simulink library "IOBlock_Library_TTC580"  (R2021a)
settings: Solver=ode45  StartTime=0.0  StopTime=10.0  RelTol=1e-3
PreLoadFcn:
  | addpath(genpath(fileparts(which('IOBlock_Library_TTC580'))));
  | %addpath(genpath(fileparts(which('IOBlock_Library_TTC580.mdl'))))
  | try
  | addpath(genpath([fileparts(which('IOBlock_Library_TTC580')),'\..\DBC_Importer']));
  | addpath(genpath([fileparts(which('IOBlock_Library_TTC580')),'\..\EEPROM_Importer']));
  | addpath(genpath([fileparts(which('IOBlock_Library_TTC580')),'\..\UserDoc']));
  | catch
  | warning('IOBlock_Library_TTC580: add path to DBC_Importer and EEPROM_Importer manually');
  | end
  | try
  | if exist('..\CustomPackage\scripts\OpenAllPackages.m','file')
  |      run('..\CustomPackage\scripts\OpenAllPackages.m'); %always available, ggf. empty
  | end
  | catch
  | warning('A problem occurred opening automatically the CustomPackage. Please open libraries manually');
  | end
  | try
  | set_param(0,'EditorSmartEditingHotParam','off');
  | catch
  | warning('Simlink preferences for ''Edit key parameter when adding new blocks'' needs to be unchecked manually');
  | end
undefined symbols (not defined in the file or in its folder): ADC_Absolute_10V, ADC_Absolute_32V, ADC_Absolute_5V, ADC_BoardTemp, ADC_ChannelInit, ADC_Current, ADC_Get, ADC_K15_, ADC_Ratiometric_10V, ADC_Ratiometric_5V, ADC_Resistive, ADC_SensorSupply, ADC_UBAT, bit_packing, bit_unpacking, CAN_ConfigMsg, compare2error, compare2FET_PROT_REENABLE, crc32_calc_intern, CRC32_EEPROM_Read, CRC32_EEPROM_Write, DIAG_EnterSafestate, DIAG_Status, DIAG_Status_internal, EEPROM_Mirror, EEPROM_Read, EEPROM_Read_OffsetIn, EEPROM_Read_Raw, EEPROM_Write, EEPROM_Write_OffsetIn, EEPROM_Write_Raw, EnterSafestate, FPU_Handler, Get_DI, Get_DI_VarThreshold, Get_K15_, Get_Pulse_Freq_Curr, Get_Pulse_Freq_Volt, Get_WakeUp, GetDateAndTime, IO_ADC_ResetProtection, IO_Blk_Lib_TTC500, IO_CAN_ReadMsg, IO_CAN_WriteMsg, IO_DI_Get, IO_DI_Init, IO_DI_Init_Var, IO_DO_GetCur, IO_DO_GetVoltage, IO_DO_Init, IO_DO_ResetProtection, IO_DO_Set, IO_Driver_GetSerialNumber, IO_Driver_GetVersionOfDriver, IO_Driver_GetVersionOfFPGA, IO_EEPROM_GetStatus, IO_EEPROM_Init, IO_EEPROM_Read_raw, IO_EEPROM_Write, IO_EEPROM_Write_OffsetIn ... (+73)
libraries: simulink x43
(part 16 of 18)

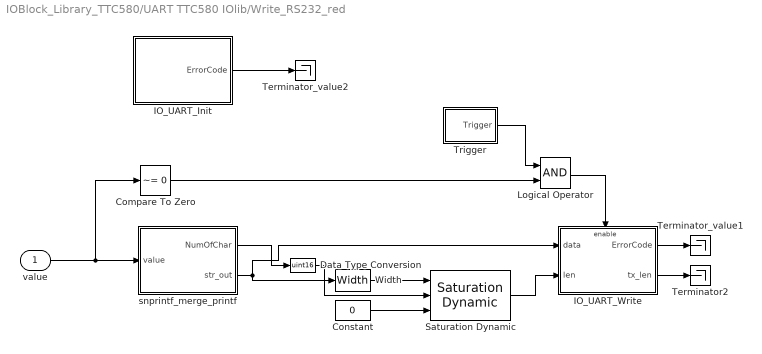
== system IOBlock_Library_TTC580/UART TTC580 IOlib/Write_RS232_red ==
  value : Inport
  Compare To Zero : simulink/Logic and Bit Operations/Compare To Zero  relop=~=  OutDataTypeStr=boolean
  Constant : Constant  Value=0  OutDataTypeStr=uint16
  Data Type Conversion : DataTypeConversion  OutDataTypeStr=uint16
  IO_UART_Init : Subsystem  LoadFcn=|  mask(IO_UART_Init_Code){SampleTime=-1, ttlib=IO_Blk_Lib_TTC500, ttDescription=IO_UART_Init, tt_iolib_version=0.25, baudrate=115200, dbits='8', par='IO_UART_PARITY_NONE', sbits='1'}
      | try
      | %
      | %Upgrade Information - standard BEGIN
      | new_color = 'blue';
      | new_ver = '0.25';
      | act_ver = get_param(gcb,'tt_iolib_version');
      | if not(strcmp(act_ver,new_ver))
      |     disp(['Upgrade block: ',gcb,char(10),'       Version: ',act_ver,' to ',new_ver]);
      |     %switch - case for specific upgrade information e.g. additional parameter required 
      |     %Change appearance and version information
      |     set_param(gcb,'ForegroundColor',new_color);
      |     set_param(gcb,'tt_iolib_version',new_ver);
      | end
      | %Upgrade Information - standard END
      | catch
      | %Standard catch section BEGIN
      | errordlg('An error occurred in a callback of the TTC580-BlockLib. Please open the Diagnostic Viewer for further details');
      | disp(' ');
      | disp('------------------------------------------------------------');
      | disp('An error occurred in a callback of the TTC580-BlockLib.');
      | disp(['Please check the parameters in the mask of ',gcb]);
      | disp('If you do not encounter any violations, then please '); 
      | disp('copy the following lines and report this to support@ttcontrol.com ');
      | disp('<< begin of error message dump >>');
      | disp(['Version of TTC580-BlockLib: ', get_param(gcb,'tt_iolib_version')]);
      | disp(get_param(gcb,'ttDescription'));
      | disp(gcb);
      | x=lasterror;disp(x.message);
      | disp(get_param(gcb,'MaskValues'));
      | disp(version);
      | disp(computer);
      | disp('<< end of error message dump >>');
      | disp('------------------------------------------------------------');
      | disp(' ');
      | %Standard catch section END
      | end
      mask help: Initialization of the UART communication driver.
      mask init:
      | %
      settings: CopyFcn=%deleted
      mask Help: No further help available for this block
      mask Callback baudrate: %
      mask Callback dbits: %
      mask Callback par: %
      mask Callback sbits: %
  IO_UART_Write : Subsystem  LoadFcn=|  mask(IO_UART_Write_Code){SampleTime=-1, ttlib=IO_Blk_Lib_TTC500, ttDescription=IO_UART_Write, tt_iolib_version=0.25}
      | try
      | %
      | %Upgrade Information - standard BEGIN
      | new_color = 'blue';
      | new_ver = '0.25';
      | act_ver = get_param(gcb,'tt_iolib_version');
      | if not(strcmp(act_ver,new_ver))
      |     disp(['Upgrade block: ',gcb,char(10),'       Version: ',act_ver,' to ',new_ver]);
      |     %switch - case for specific upgrade information e.g. additional parameter required 
      |     %Change appearance and version information
      |     set_param(gcb,'ForegroundColor',new_color);
      |     set_param(gcb,'tt_iolib_version',new_ver);
      | end
      | %Upgrade Information - standard END
      | catch
      | %Standard catch section BEGIN
      | errordlg('An error occurred in a callback of the TTC580-BlockLib. Please open the Diagnostic Viewer for further details');
      | disp(' ');
      | disp('------------------------------------------------------------');
      | disp('An error occurred in a callback of the TTC580-BlockLib.');
      | disp(['Please check the parameters in the mask of ',gcb]);
      | disp('If you do not encounter any violations, then please '); 
      | disp('copy the following lines and report this to support@ttcontrol.com ');
      | disp('<< begin of error message dump >>');
      | disp(['Version of TTC580-BlockLib: ', get_param(gcb,'tt_iolib_version')]);
      | disp(get_param(gcb,'ttDescription'));
      | disp(gcb);
      | x=lasterror;disp(x.message);
      | disp(get_param(gcb,'MaskValues'));
      | disp(version);
      | disp(computer);
      | disp('<< end of error message dump >>');
      | disp('------------------------------------------------------------');
      | disp(' ');
      | %Standard catch section END
      | end
      mask help: Write data to serial interface.
      mask init:
      | %
      settings: CopyFcn=%deleted  RTWSystemCode=Inline
      mask Help: No further help available for this block
  Logical Operator : Logic  AllPortsSameDT=off  OutDataTypeStr=boolean
  Saturation Dynamic : simulink/Discontinuities/Saturation Dynamic  OutMin=[]  OutMax=[]  OutDataTypeStr=uint16  OutputDataTypeScalingMode=uint16  OutDataType=fixdt(1, 16)  OutScaling=2^-10  DoSatur=off
  Terminator2 : Terminator
  Terminator_value1 : Terminator
  Terminator_value2 : Terminator
  Trigger : Subsystem  mask(Derate Trigger){derate=derate_val}
      mask help: derate "n": every n-th cylce a trigger is submitted
  Width : Width  DataType=uint16
  snprintf_merge_printf : Subsystem  LoadFcn=|  mask(snprintf_merge_printf_Code){SampleTime=-1, ttlib=IO_Blk_Lib_TTC500, ttDescription=snprintf_merge_printf, tt_iolib_version=0.25, max_size=80, Comment=['\033[0;31m',Comment,'\033[0m']}
      | try
      | %
      | %Upgrade Information - standard BEGIN
      | new_color = 'blue';
      | new_ver = '0.25';
      | act_ver = get_param(gcb,'tt_iolib_version');
      | if not(strcmp(act_ver,new_ver))
      |     disp(['Upgrade block: ',gcb,char(10),'       Version: ',act_ver,' to ',new_ver]);
      |     %switch - case for specific upgrade information e.g. additional parameter required 
      |     %Change appearance and version information
      |     set_param(gcb,'ForegroundColor',new_color);
      |     set_param(gcb,'tt_iolib_version',new_ver);
      | end
      | %Upgrade Information - standard END
      | catch
      | %Standard catch section BEGIN
      | errordlg('An error occurred in a callback of the TTC580-BlockLib. Please open the Diagnostic Viewer for further details');
      | disp(' ');
      | disp('------------------------------------------------------------');
      | disp('An error occurred in a callback of the TTC580-BlockLib.');
      | disp(['Please check the parameters in the mask of ',gcb]);
      | disp('If you do not encounter any violations, then please '); 
      | disp('copy the following lines and report this to support@ttcontrol.com ');
      | disp('<< begin of error message dump >>');
      | disp(['Version of TTC580-BlockLib: ', get_param(gcb,'tt_iolib_version')]);
      | disp(get_param(gcb,'ttDescription'));
      | disp(gcb);
      | x=lasterror;disp(x.message);
      | disp(get_param(gcb,'MaskValues'));
      | disp(version);
      | disp(computer);
      | disp('<< end of error message dump >>');
      | disp('------------------------------------------------------------');
      | disp(' ');
      | %Standard catch section END
      | end
      mask help:
      | The C library function snprintf sends formatted output to a string with maximum length of n characters.
      | This snprintf implementation adds LF and reset cursor information the way that the printf implementation did it before
      mask init:
      | %
      settings: CopyFcn=%deleted
      mask Help: No further help available for this block
      mask Callback max_size: %
      mask Callback Comment: %
  wires:
  Data Type Conversion/1 -> Saturation Dynamic/2
  IO_UART_Write/1(ErrorCode) -> Terminator_value1/1
  Constant/1 -> Saturation Dynamic/3
  value/1 -> snprintf_merge_printf/1(value), Compare To Zero/1
  snprintf_merge_printf/1(NumOfChar) -> Data Type Conversion/1
  Width/1 -> Saturation Dynamic/1
  IO_UART_Init/1(ErrorCode) -> Terminator_value2/1
  Saturation Dynamic/1 -> IO_UART_Write/2(len)
  snprintf_merge_printf/2(str_out) -> IO_UART_Write/1(data), Width/1
  IO_UART_Write/2(tx_len) -> Terminator2/1
  Trigger/1(Trigger) -> Logical Operator/1
  Compare To Zero/1 -> Logical Operator/2
  Logical Operator/1 -> IO_UART_Write/Enable

== system IOBlock_Library_TTC580/ADC Blocks TTC580 IOlib/ADC_Absolute_10V/ADC_ChannelInit ==
  ADC_ChannelInit_s : S-Function  FunctionName=ADC_ChannelInit_s  Parameters=SampleTime,adc_channel,adc_type,range,pupd,sensor_supply,safety_conf  SFunctionDeploymentMode=off  EnableBusSupport=off
  ErrorCode : Outport  VectorParamsAs1DForOutWhenUnconnected=off
  wires:
  ADC_ChannelInit_s/1 -> ErrorCode/1

== system IOBlock_Library_TTC580/ADC Blocks TTC580 IOlib/ADC_Absolute_10V/ADC_Get ==
  ADC_Get_s : S-Function  FunctionName=ADC_Get_s  Parameters=SampleTime,adc_channel  SFunctionDeploymentMode=off  EnableBusSupport=off
  ErrorCode : Outport  VectorParamsAs1DForOutWhenUnconnected=off
  adc_value : Outport  Port=2  VectorParamsAs1DForOutWhenUnconnected=off
  fresh : Outport  Port=3  VectorParamsAs1DForOutWhenUnconnected=off
  wires:
  ADC_Get_s/3 -> fresh/1
  ADC_Get_s/2 -> adc_value/1
  ADC_Get_s/1 -> ErrorCode/1

== system IOBlock_Library_TTC580/ADC Blocks TTC580 IOlib/ADC_Absolute_32V/ADC_ChannelInit ==
  ADC_ChannelInit_s : S-Function  FunctionName=ADC_ChannelInit_s  Parameters=SampleTime,adc_channel,adc_type,range,pupd,sensor_supply,safety_conf  SFunctionDeploymentMode=off  EnableBusSupport=off
  ErrorCode : Outport  VectorParamsAs1DForOutWhenUnconnected=off
  wires:
  ADC_ChannelInit_s/1 -> ErrorCode/1

== system IOBlock_Library_TTC580/ADC Blocks TTC580 IOlib/ADC_Absolute_32V/ADC_Get ==
  ADC_Get_s : S-Function  FunctionName=ADC_Get_s  Parameters=SampleTime,adc_channel  SFunctionDeploymentMode=off  EnableBusSupport=off
  ErrorCode : Outport  VectorParamsAs1DForOutWhenUnconnected=off
  adc_value : Outport  Port=2  VectorParamsAs1DForOutWhenUnconnected=off
  fresh : Outport  Port=3  VectorParamsAs1DForOutWhenUnconnected=off
  wires:
  ADC_Get_s/3 -> fresh/1
  ADC_Get_s/2 -> adc_value/1
  ADC_Get_s/1 -> ErrorCode/1

== system IOBlock_Library_TTC580/ADC Blocks TTC580 IOlib/ADC_Absolute_5V/ADC_ChannelInit ==
  ADC_ChannelInit_s : S-Function  FunctionName=ADC_ChannelInit_s  Parameters=SampleTime,adc_channel,adc_type,range,pupd,sensor_supply,safety_conf  SFunctionDeploymentMode=off  EnableBusSupport=off
  ErrorCode : Outport  VectorParamsAs1DForOutWhenUnconnected=off
  wires:
  ADC_ChannelInit_s/1 -> ErrorCode/1

== system IOBlock_Library_TTC580/ADC Blocks TTC580 IOlib/ADC_Absolute_5V/ADC_Get ==
  ADC_Get_s : S-Function  FunctionName=ADC_Get_s  Parameters=SampleTime,adc_channel  SFunctionDeploymentMode=off  EnableBusSupport=off
  ErrorCode : Outport  VectorParamsAs1DForOutWhenUnconnected=off
  adc_value : Outport  Port=2  VectorParamsAs1DForOutWhenUnconnected=off
  fresh : Outport  Port=3  VectorParamsAs1DForOutWhenUnconnected=off
  wires:
  ADC_Get_s/3 -> fresh/1
  ADC_Get_s/2 -> adc_value/1
  ADC_Get_s/1 -> ErrorCode/1

== system IOBlock_Library_TTC580/ADC Blocks TTC580 IOlib/ADC_BoardTemp/ADC_ChannelInit ==
  ADC_ChannelInit_s : S-Function  FunctionName=ADC_ChannelInit_s  Parameters=SampleTime,adc_channel,adc_type,range,pupd,sensor_supply,safety_conf  SFunctionDeploymentMode=off  EnableBusSupport=off
  ErrorCode : Outport  VectorParamsAs1DForOutWhenUnconnected=off
  wires:
  ADC_ChannelInit_s/1 -> ErrorCode/1

== system IOBlock_Library_TTC580/ADC Blocks TTC580 IOlib/ADC_BoardTemp/ADC_Get ==
  ADC_Get_s : S-Function  FunctionName=ADC_Get_s  Parameters=SampleTime,adc_channel  SFunctionDeploymentMode=off  EnableBusSupport=off
  ErrorCode : Outport  VectorParamsAs1DForOutWhenUnconnected=off
  adc_value : Outport  Port=2  VectorParamsAs1DForOutWhenUnconnected=off
  fresh : Outport  Port=3  VectorParamsAs1DForOutWhenUnconnected=off
  wires:
  ADC_Get_s/1 -> ErrorCode/1
  ADC_Get_s/2 -> adc_value/1
  ADC_Get_s/3 -> fresh/1

== system IOBlock_Library_TTC580/ADC Blocks TTC580 IOlib/ADC_Current/ADC_ChannelInit ==
  ADC_ChannelInit_s : S-Function  FunctionName=ADC_ChannelInit_s  Parameters=SampleTime,adc_channel,adc_type,range,pupd,sensor_supply,safety_conf  SFunctionDeploymentMode=off  EnableBusSupport=off
  ErrorCode : Outport  VectorParamsAs1DForOutWhenUnconnected=off
  wires:
  ADC_ChannelInit_s/1 -> ErrorCode/1

== system IOBlock_Library_TTC580/ADC Blocks TTC580 IOlib/ADC_Current/ADC_Get ==
  ADC_Get_s : S-Function  FunctionName=ADC_Get_s  Parameters=SampleTime,adc_channel  SFunctionDeploymentMode=off  EnableBusSupport=off
  ErrorCode : Outport  VectorParamsAs1DForOutWhenUnconnected=off
  adc_value : Outport  Port=2  VectorParamsAs1DForOutWhenUnconnected=off
  fresh : Outport  Port=3  VectorParamsAs1DForOutWhenUnconnected=off
  wires:
  ADC_Get_s/3 -> fresh/1
  ADC_Get_s/2 -> adc_value/1
  ADC_Get_s/1 -> ErrorCode/1

== system IOBlock_Library_TTC580/ADC Blocks TTC580 IOlib/ADC_Current/IO_ADC_ResetProtection ==
  Trigger : TriggerPort  VariantControl=(inherit)
  IO_ADC_ResetProtection_s : S-Function  FunctionName=IO_ADC_ResetProtection_s  Parameters=SampleTime,adc_channel  SFunctionDeploymentMode=off  EnableBusSupport=off
  ErrorCode : Outport  VectorParamsAs1DForOutWhenUnconnected=off
  reset_cnt : Outport  Port=2  VectorParamsAs1DForOutWhenUnconnected=off
  wires:
  IO_ADC_ResetProtection_s/2 -> reset_cnt/1
  IO_ADC_ResetProtection_s/1 -> ErrorCode/1

== system IOBlock_Library_TTC580/ADC Blocks TTC580 IOlib/ADC_Current/compare2FET_PROT_REENABLE ==
  Errorcode : Inport  OutDataTypeStr=uint16
  compare2error_s : S-Function  FunctionName=compare2error_s  Parameters=SampleTime,define  SFunctionDeploymentMode=off  EnableBusSupport=off
  b_compare : Outport  VectorParamsAs1DForOutWhenUnconnected=off
  wires:
  Errorcode/1 -> compare2error_s/1
  compare2error_s/1 -> b_compare/1

== system IOBlock_Library_TTC580/ADC Blocks TTC580 IOlib/ADC_K15_/ADC_ChannelInit ==
  ADC_ChannelInit_s : S-Function  FunctionName=ADC_ChannelInit_s  Parameters=SampleTime,adc_channel,adc_type,range,pupd,sensor_supply,safety_conf  SFunctionDeploymentMode=off  EnableBusSupport=off
  ErrorCode : Outport  VectorParamsAs1DForOutWhenUnconnected=off
  wires:
  ADC_ChannelInit_s/1 -> ErrorCode/1

== system IOBlock_Library_TTC580/ADC Blocks TTC580 IOlib/ADC_K15_/ADC_Get ==
  ADC_Get_s : S-Function  FunctionName=ADC_Get_s  Parameters=SampleTime,adc_channel  SFunctionDeploymentMode=off  EnableBusSupport=off
  ErrorCode : Outport  VectorParamsAs1DForOutWhenUnconnected=off
  adc_value : Outport  Port=2  VectorParamsAs1DForOutWhenUnconnected=off
  fresh : Outport  Port=3  VectorParamsAs1DForOutWhenUnconnected=off
  wires:
  ADC_Get_s/1 -> ErrorCode/1
  ADC_Get_s/2 -> adc_value/1
  ADC_Get_s/3 -> fresh/1

== system IOBlock_Library_TTC580/ADC Blocks TTC580 IOlib/ADC_Ratiometric_10V/ADC_ChannelInit ==
  ADC_ChannelInit_s : S-Function  FunctionName=ADC_ChannelInit_s  Parameters=SampleTime,adc_channel,adc_type,range,pupd,sensor_supply,safety_conf  SFunctionDeploymentMode=off  EnableBusSupport=off
  ErrorCode : Outport  VectorParamsAs1DForOutWhenUnconnected=off
  wires:
  ADC_ChannelInit_s/1 -> ErrorCode/1

== system IOBlock_Library_TTC580/ADC Blocks TTC580 IOlib/ADC_Ratiometric_10V/ADC_Get ==
  ADC_Get_s : S-Function  FunctionName=ADC_Get_s  Parameters=SampleTime,adc_channel  SFunctionDeploymentMode=off  EnableBusSupport=off
  ErrorCode : Outport  VectorParamsAs1DForOutWhenUnconnected=off
  adc_value : Outport  Port=2  VectorParamsAs1DForOutWhenUnconnected=off
  fresh : Outport  Port=3  VectorParamsAs1DForOutWhenUnconnected=off
  wires:
  ADC_Get_s/1 -> ErrorCode/1
  ADC_Get_s/2 -> adc_value/1
  ADC_Get_s/3 -> fresh/1

== system IOBlock_Library_TTC580/ADC Blocks TTC580 IOlib/ADC_Ratiometric_10V/POWER_Set_Init ==
  POWER_Set_Init_s : S-Function  FunctionName=POWER_Set_Init_s  Parameters=SampleTime,pin,mode  SFunctionDeploymentMode=off  EnableBusSupport=off
  ErrorCode : Outport  VectorParamsAs1DForOutWhenUnconnected=off
  wires:
  POWER_Set_Init_s/1 -> ErrorCode/1

== system IOBlock_Library_TTC580/ADC Blocks TTC580 IOlib/ADC_Ratiometric_5V/ADC_ChannelInit ==
  ADC_ChannelInit_s : S-Function  FunctionName=ADC_ChannelInit_s  Parameters=SampleTime,adc_channel,adc_type,range,pupd,sensor_supply,safety_conf  SFunctionDeploymentMode=off  EnableBusSupport=off
  ErrorCode : Outport  VectorParamsAs1DForOutWhenUnconnected=off
  wires:
  ADC_ChannelInit_s/1 -> ErrorCode/1

== system IOBlock_Library_TTC580/ADC Blocks TTC580 IOlib/ADC_Ratiometric_5V/ADC_Get ==
  ADC_Get_s : S-Function  FunctionName=ADC_Get_s  Parameters=SampleTime,adc_channel  SFunctionDeploymentMode=off  EnableBusSupport=off
  ErrorCode : Outport  VectorParamsAs1DForOutWhenUnconnected=off
  adc_value : Outport  Port=2  VectorParamsAs1DForOutWhenUnconnected=off
  fresh : Outport  Port=3  VectorParamsAs1DForOutWhenUnconnected=off
  wires:
  ADC_Get_s/1 -> ErrorCode/1
  ADC_Get_s/2 -> adc_value/1
  ADC_Get_s/3 -> fresh/1

== system IOBlock_Library_TTC580/ADC Blocks TTC580 IOlib/ADC_Ratiometric_5V/POWER_Set_Init ==
  POWER_Set_Init_s : S-Function  FunctionName=POWER_Set_Init_s  Parameters=SampleTime,pin,mode  SFunctionDeploymentMode=off  EnableBusSupport=off
  ErrorCode : Outport  VectorParamsAs1DForOutWhenUnconnected=off
  wires:
  POWER_Set_Init_s/1 -> ErrorCode/1

== system IOBlock_Library_TTC580/ADC Blocks TTC580 IOlib/ADC_Resistive/ADC_ChannelInit ==
  ADC_ChannelInit_s : S-Function  FunctionName=ADC_ChannelInit_s  Parameters=SampleTime,adc_channel,adc_type,range,pupd,sensor_supply,safety_conf  SFunctionDeploymentMode=off  EnableBusSupport=off
  ErrorCode : Outport  VectorParamsAs1DForOutWhenUnconnected=off
  wires:
  ADC_ChannelInit_s/1 -> ErrorCode/1

== system IOBlock_Library_TTC580/ADC Blocks TTC580 IOlib/ADC_Resistive/ADC_Get ==
  ADC_Get_s : S-Function  FunctionName=ADC_Get_s  Parameters=SampleTime,adc_channel  SFunctionDeploymentMode=off  EnableBusSupport=off
  ErrorCode : Outport  VectorParamsAs1DForOutWhenUnconnected=off
  adc_value : Outport  Port=2  VectorParamsAs1DForOutWhenUnconnected=off
  fresh : Outport  Port=3  VectorParamsAs1DForOutWhenUnconnected=off
  wires:
  ADC_Get_s/3 -> fresh/1
  ADC_Get_s/2 -> adc_value/1
  ADC_Get_s/1 -> ErrorCode/1

== system IOBlock_Library_TTC580/ADC Blocks TTC580 IOlib/ADC_SensorSupply/ADC_ChannelInit ==
  ADC_ChannelInit_s : S-Function  FunctionName=ADC_ChannelInit_s  Parameters=SampleTime,adc_channel,adc_type,range,pupd,sensor_supply,safety_conf  SFunctionDeploymentMode=off  EnableBusSupport=off
  ErrorCode : Outport  VectorParamsAs1DForOutWhenUnconnected=off
  wires:
  ADC_ChannelInit_s/1 -> ErrorCode/1

== system IOBlock_Library_TTC580/ADC Blocks TTC580 IOlib/ADC_SensorSupply/ADC_Get ==
  ADC_Get_s : S-Function  FunctionName=ADC_Get_s  Parameters=SampleTime,adc_channel  SFunctionDeploymentMode=off  EnableBusSupport=off
  ErrorCode : Outport  VectorParamsAs1DForOutWhenUnconnected=off
  adc_value : Outport  Port=2  VectorParamsAs1DForOutWhenUnconnected=off
  fresh : Outport  Port=3  VectorParamsAs1DForOutWhenUnconnected=off
  wires:
  ADC_Get_s/3 -> fresh/1
  ADC_Get_s/2 -> adc_value/1
  ADC_Get_s/1 -> ErrorCode/1

== system IOBlock_Library_TTC580/ADC Blocks TTC580 IOlib/ADC_UBAT/ADC_ChannelInit ==
  ADC_ChannelInit_s : S-Function  FunctionName=ADC_ChannelInit_s  Parameters=SampleTime,adc_channel,adc_type,range,pupd,sensor_supply,safety_conf  SFunctionDeploymentMode=off  EnableBusSupport=off
  ErrorCode : Outport  VectorParamsAs1DForOutWhenUnconnected=off
  wires:
  ADC_ChannelInit_s/1 -> ErrorCode/1

== system IOBlock_Library_TTC580/ADC Blocks TTC580 IOlib/ADC_UBAT/ADC_Get ==
  ADC_Get_s : S-Function  FunctionName=ADC_Get_s  Parameters=SampleTime,adc_channel  SFunctionDeploymentMode=off  EnableBusSupport=off
  ErrorCode : Outport  VectorParamsAs1DForOutWhenUnconnected=off
  adc_value : Outport  Port=2  VectorParamsAs1DForOutWhenUnconnected=off
  fresh : Outport  Port=3  VectorParamsAs1DForOutWhenUnconnected=off
  wires:
  ADC_Get_s/3 -> fresh/1
  ADC_Get_s/2 -> adc_value/1
  ADC_Get_s/1 -> ErrorCode/1

== system IOBlock_Library_TTC580/CAN  Blocks TTC580 IOlib/ReadMsg_CAN/CAN_ConfigMsg ==
  CAN_ConfigMsg_s : S-Function  FunctionName=CAN_ConfigMsg_s  Parameters=SampleTime,channel,mode,id_format,id,ac_mask  SFunctionDeploymentMode=off  EnableBusSupport=off
  ErrorCode : Outport  VectorParamsAs1DForOutWhenUnconnected=off
  handle : Outport  Port=2  VectorParamsAs1DForOutWhenUnconnected=off
  wires:
  CAN_ConfigMsg_s/2 -> handle/1
  CAN_ConfigMsg_s/1 -> ErrorCode/1

== system IOBlock_Library_TTC580/CAN  Blocks TTC580 IOlib/ReadMsg_CAN/IO_CAN_ReadMsg ==
  handle : Inport
  IO_CAN_ReadMsg_s : S-Function  FunctionName=IO_CAN_ReadMsg_s  Parameters=SampleTime  SFunctionDeploymentMode=off  EnableBusSupport=off
  ErrorCode : Outport  VectorParamsAs1DForOutWhenUnconnected=off
  buffer_data : Outport  Port=2  VectorParamsAs1DForOutWhenUnconnected=off
  buffer_length : Outport  Port=3  VectorParamsAs1DForOutWhenUnconnected=off
  buffer_id_format : Outport  Port=4  VectorParamsAs1DForOutWhenUnconnected=off
  buffer_id : Outport  Port=5  VectorParamsAs1DForOutWhenUnconnected=off
  wires:
  IO_CAN_ReadMsg_s/5 -> buffer_id/1
  IO_CAN_ReadMsg_s/4 -> buffer_id_format/1
  IO_CAN_ReadMsg_s/3 -> buffer_length/1
  IO_CAN_ReadMsg_s/2 -> buffer_data/1
  IO_CAN_ReadMsg_s/1 -> ErrorCode/1
  handle/1 -> IO_CAN_ReadMsg_s/1

== system IOBlock_Library_TTC580/CAN  Blocks TTC580 IOlib/ReadMsg_CAN_derated/CAN_ConfigMsg ==
  CAN_ConfigMsg_s : S-Function  FunctionName=CAN_ConfigMsg_s  Parameters=SampleTime,channel,mode,id_format,id,ac_mask  SFunctionDeploymentMode=off  EnableBusSupport=off
  ErrorCode : Outport  VectorParamsAs1DForOutWhenUnconnected=off
  handle : Outport  Port=2  VectorParamsAs1DForOutWhenUnconnected=off
  wires:
  CAN_ConfigMsg_s/1 -> ErrorCode/1
  CAN_ConfigMsg_s/2 -> handle/1

== system IOBlock_Library_TTC580/CAN  Blocks TTC580 IOlib/ReadMsg_CAN_derated/IO_CAN_ReadMsg_x ==
  handle : Inport
  Enable : EnablePort
  IO_CAN_ReadMsg_s : S-Function  FunctionName=IO_CAN_ReadMsg_s  Parameters=SampleTime  SFunctionDeploymentMode=off  EnableBusSupport=off
  debounce_alternate : Subsystem
  ErrorCode : Outport  InitialOutput=16 %IO_E_STARTUP, just in case not debounced correctly  VectorParamsAs1DForOutWhenUnconnected=off
  buffer_data : Outport  Port=2  VectorParamsAs1DForOutWhenUnconnected=off
  buffer_length : Outport  Port=3  VectorParamsAs1DForOutWhenUnconnected=off
  buffer_id_format : Outport  Port=4  VectorParamsAs1DForOutWhenUnconnected=off
  buffer_id : Outport  Port=5  VectorParamsAs1DForOutWhenUnconnected=off
  wires:
  debounce_alternate/1(Out) -> ErrorCode/1
  handle/1 -> IO_CAN_ReadMsg_s/1
  IO_CAN_ReadMsg_s/1 -> debounce_alternate/1(In)
  IO_CAN_ReadMsg_s/2 -> buffer_data/1
  IO_CAN_ReadMsg_s/3 -> buffer_length/1
  IO_CAN_ReadMsg_s/4 -> buffer_id_format/1
  IO_CAN_ReadMsg_s/5 -> buffer_id/1

== system IOBlock_Library_TTC580/CAN  Blocks TTC580 IOlib/ReadMsg_CAN_derated/Trigger ==
  Compare To Constant : simulink/Logic and Bit Operations/Compare To Constant  relop===  const=0  OutDataTypeStr=boolean  ZeroCross=off
  Counter Limited : simulink/Sources/Counter Limited  uplimit=max(derate - 1,0)  tsamp=-1
  Trigger : Outport  VectorParamsAs1DForOutWhenUnconnected=off
  wires:
  Compare To Constant/1 -> Trigger/1
  Counter Limited/1 -> Compare To Constant/1

== system IOBlock_Library_TTC580/CAN  Blocks TTC580 IOlib/WriteMsg_CAN/CAN_ConfigMsg ==
  CAN_ConfigMsg_s : S-Function  FunctionName=CAN_ConfigMsg_s  Parameters=SampleTime,channel,mode,id_format,id,ac_mask  SFunctionDeploymentMode=off  EnableBusSupport=off
  ErrorCode : Outport  VectorParamsAs1DForOutWhenUnconnected=off
  handle : Outport  Port=2  VectorParamsAs1DForOutWhenUnconnected=off
  wires:
  CAN_ConfigMsg_s/2 -> handle/1
  CAN_ConfigMsg_s/1 -> ErrorCode/1

== system IOBlock_Library_TTC580/CAN  Blocks TTC580 IOlib/WriteMsg_CAN/IO_CAN_WriteMsg ==
  handle : Inport
  buffer_data : Inport  Port=2
  buffer_length : Inport  Port=3
  buffer_id_format : Inport  Port=4
  buffer_id : Inport  Port=5
  IO_CAN_WriteMsg_s : S-Function  FunctionName=IO_CAN_WriteMsg_s  Parameters=SampleTime  SFunctionDeploymentMode=off  EnableBusSupport=off
  ErrorCode : Outport  VectorParamsAs1DForOutWhenUnconnected=off
  wires:
  IO_CAN_WriteMsg_s/1 -> ErrorCode/1
  buffer_id/1 -> IO_CAN_WriteMsg_s/5
  buffer_id_format/1 -> IO_CAN_WriteMsg_s/4
  buffer_length/1 -> IO_CAN_WriteMsg_s/3
  buffer_data/1 -> IO_CAN_WriteMsg_s/2
  handle/1 -> IO_CAN_WriteMsg_s/1

== system IOBlock_Library_TTC580/CAN  Blocks TTC580 IOlib/WriteMsg_CAN_derated/CAN_ConfigMsg ==
  CAN_ConfigMsg_s : S-Function  FunctionName=CAN_ConfigMsg_s  Parameters=SampleTime,channel,mode,id_format,id,ac_mask  SFunctionDeploymentMode=off  EnableBusSupport=off
  ErrorCode : Outport  VectorParamsAs1DForOutWhenUnconnected=off
  handle : Outport  Port=2  VectorParamsAs1DForOutWhenUnconnected=off
  wires:
  CAN_ConfigMsg_s/2 -> handle/1
  CAN_ConfigMsg_s/1 -> ErrorCode/1

== system IOBlock_Library_TTC580/CAN  Blocks TTC580 IOlib/WriteMsg_CAN_derated/IO_CAN_WriteMsg_x ==
  handle : Inport
  buffer_data : Inport  Port=2
  buffer_length : Inport  Port=3
  buffer_id_format : Inport  Port=4
  buffer_id : Inport  Port=5
  Enable : EnablePort
  IO_CAN_WriteMsg_s : S-Function  FunctionName=IO_CAN_WriteMsg_s  Parameters=SampleTime  SFunctionDeploymentMode=off  EnableBusSupport=off
  ErrorCode : Outport  InitialOutput=16 %IO_E_STARTUP, just in case not debounced correctly  VectorParamsAs1DForOutWhenUnconnected=off
  wires:
  IO_CAN_WriteMsg_s/1 -> ErrorCode/1
  buffer_id/1 -> IO_CAN_WriteMsg_s/5
  buffer_id_format/1 -> IO_CAN_WriteMsg_s/4
  buffer_length/1 -> IO_CAN_WriteMsg_s/3
  buffer_data/1 -> IO_CAN_WriteMsg_s/2
  handle/1 -> IO_CAN_WriteMsg_s/1

== system IOBlock_Library_TTC580/CAN  Blocks TTC580 IOlib/WriteMsg_CAN_derated/Trigger ==
  Compare To Constant : simulink/Logic and Bit Operations/Compare To Constant  relop===  const=0  OutDataTypeStr=boolean  ZeroCross=off
  Counter Limited : simulink/Sources/Counter Limited  uplimit=max(derate - 1,0)  tsamp=-1
  Trigger : Outport  VectorParamsAs1DForOutWhenUnconnected=off
  wires:
  Compare To Constant/1 -> Trigger/1
  Counter Limited/1 -> Compare To Constant/1

== system IOBlock_Library_TTC580/DIO Blocks TTC580 IOlib/Get_DI/IO_DI_Get ==
  IO_DI_Get_s : S-Function  FunctionName=IO_DI_Get_s  Parameters=SampleTime,di_channel  SFunctionDeploymentMode=off  EnableBusSupport=off
  ErrorCode : Outport  VectorParamsAs1DForOutWhenUnconnected=off
  di_value : Outport  Port=2  VectorParamsAs1DForOutWhenUnconnected=off
  wires:
  IO_DI_Get_s/1 -> ErrorCode/1
  IO_DI_Get_s/2 -> di_value/1

== system IOBlock_Library_TTC580/DIO Blocks TTC580 IOlib/Get_DI/IO_DI_Init ==
  IO_DI_Init_s : S-Function  FunctionName=IO_DI_Init_s  Parameters=SampleTime,di_channel,pupd,limits  SFunctionDeploymentMode=off  EnableBusSupport=off
  ErrorCode : Outport  VectorParamsAs1DForOutWhenUnconnected=off
  wires:
  IO_DI_Init_s/1 -> ErrorCode/1

== system IOBlock_Library_TTC580/DIO Blocks TTC580 IOlib/Get_DI_VarThreshold/IO_DI_Get ==
  IO_DI_Get_s : S-Function  FunctionName=IO_DI_Get_s  Parameters=SampleTime,di_channel  SFunctionDeploymentMode=off  EnableBusSupport=off
  ErrorCode : Outport  VectorParamsAs1DForOutWhenUnconnected=off
  di_value : Outport  Port=2  VectorParamsAs1DForOutWhenUnconnected=off
  wires:
  IO_DI_Get_s/2 -> di_value/1
  IO_DI_Get_s/1 -> ErrorCode/1

== system IOBlock_Library_TTC580/DIO Blocks TTC580 IOlib/Get_DI_VarThreshold/IO_DI_Init_Var ==
  IO_DI_Init_Var_s : S-Function  FunctionName=IO_DI_Init_Var_s  Parameters=SampleTime,di_channel,pupd,limits_low_thresh1,limits_low_thresh2,limits_high_thresh1,limits_high_thresh2  SFunctionDeploymentMode=off  EnableBusSupport=off
  ErrorCode : Outport  VectorParamsAs1DForOutWhenUnconnected=off
  wires:
  IO_DI_Init_Var_s/1 -> ErrorCode/1

== system IOBlock_Library_TTC580/DIO Blocks TTC580 IOlib/Get_K15_/POWER_Get ==
  POWER_Get_s : S-Function  FunctionName=POWER_Get_s  Parameters=SampleTime,pin  SFunctionDeploymentMode=off  EnableBusSupport=off
  ErrorCode : Outport  VectorParamsAs1DForOutWhenUnconnected=off
  state : Outport  Port=2  VectorParamsAs1DForOutWhenUnconnected=off
  wires:
  POWER_Get_s/2 -> state/1
  POWER_Get_s/1 -> ErrorCode/1

== system IOBlock_Library_TTC580/DIO Blocks TTC580 IOlib/Get_WakeUp/POWER_Get ==
  POWER_Get_s : S-Function  FunctionName=POWER_Get_s  Parameters=SampleTime,pin  SFunctionDeploymentMode=off  EnableBusSupport=off
  ErrorCode : Outport  VectorParamsAs1DForOutWhenUnconnected=off
  state : Outport  Port=2  VectorParamsAs1DForOutWhenUnconnected=off
  wires:
  POWER_Get_s/2 -> state/1
  POWER_Get_s/1 -> ErrorCode/1

== system IOBlock_Library_TTC580/DIO Blocks TTC580 IOlib/Set_DO_HighSide/IO_DO_Init ==
  IO_DO_Init_s : S-Function  FunctionName=IO_DO_Init_s  Parameters=SampleTime,do_channel,diagnostic,safety_conf  SFunctionDeploymentMode=off  EnableBusSupport=off
  ErrorCode : Outport  VectorParamsAs1DForOutWhenUnconnected=off
  wires:
  IO_DO_Init_s/1 -> ErrorCode/1

== system IOBlock_Library_TTC580/DIO Blocks TTC580 IOlib/Set_DO_HighSide/IO_DO_ResetProtection ==
  Trigger : TriggerPort  VariantControl=(inherit)
  IO_DO_ResetProtection_s : S-Function  FunctionName=IO_DO_ResetProtection_s  Parameters=SampleTime,do_channel  SFunctionDeploymentMode=off  EnableBusSupport=off
  ErrorCode : Outport  VectorParamsAs1DForOutWhenUnconnected=off
  reset_cnt : Outport  Port=2  VectorParamsAs1DForOutWhenUnconnected=off
  wires:
  IO_DO_ResetProtection_s/1 -> ErrorCode/1
  IO_DO_ResetProtection_s/2 -> reset_cnt/1

== system IOBlock_Library_TTC580/DIO Blocks TTC580 IOlib/Set_DO_HighSide/IO_DO_Set ==
  do_value : Inport
  IO_DO_Set_s : S-Function  FunctionName=IO_DO_Set_s  Parameters=SampleTime,do_channel  SFunctionDeploymentMode=off  EnableBusSupport=off
  ErrorCode : Outport  VectorParamsAs1DForOutWhenUnconnected=off
  wires:
  do_value/1 -> IO_DO_Set_s/1
  IO_DO_Set_s/1 -> ErrorCode/1

== system IOBlock_Library_TTC580/DIO Blocks TTC580 IOlib/Set_DO_HighSide/compare2FET_PROT_REENABLE ==
  Errorcode : Inport  OutDataTypeStr=uint16
  compare2error_s : S-Function  FunctionName=compare2error_s  Parameters=SampleTime,define  SFunctionDeploymentMode=off  EnableBusSupport=off
  b_compare : Outport  VectorParamsAs1DForOutWhenUnconnected=off
  wires:
  Errorcode/1 -> compare2error_s/1
  compare2error_s/1 -> b_compare/1

== system IOBlock_Library_TTC580/DIO Blocks TTC580 IOlib/Set_DO_HighSide_Fullfb/IO_DO_GetCur ==
  IO_DO_GetCur_s : S-Function  FunctionName=IO_DO_GetCur_s  Parameters=SampleTime,do_channel  SFunctionDeploymentMode=off  EnableBusSupport=off
  ErrorCode : Outport  VectorParamsAs1DForOutWhenUnconnected=off
  current : Outport  Port=2  VectorParamsAs1DForOutWhenUnconnected=off
  fresh : Outport  Port=3  VectorParamsAs1DForOutWhenUnconnected=off
  wires:
  IO_DO_GetCur_s/3 -> fresh/1
  IO_DO_GetCur_s/2 -> current/1
  IO_DO_GetCur_s/1 -> ErrorCode/1

== system IOBlock_Library_TTC580/DIO Blocks TTC580 IOlib/Set_DO_HighSide_Fullfb/IO_DO_GetVoltage ==
  IO_DO_GetVoltage_s : S-Function  FunctionName=IO_DO_GetVoltage_s  Parameters=SampleTime,do_channel  SFunctionDeploymentMode=off  EnableBusSupport=off
  ErrorCode : Outport  VectorParamsAs1DForOutWhenUnconnected=off
  voltage : Outport  Port=2  VectorParamsAs1DForOutWhenUnconnected=off
  fresh : Outport  Port=3  VectorParamsAs1DForOutWhenUnconnected=off
  wires:
  IO_DO_GetVoltage_s/3 -> fresh/1
  IO_DO_GetVoltage_s/2 -> voltage/1
  IO_DO_GetVoltage_s/1 -> ErrorCode/1

== system IOBlock_Library_TTC580/DIO Blocks TTC580 IOlib/Set_DO_HighSide_Fullfb/IO_DO_Init ==
  IO_DO_Init_s : S-Function  FunctionName=IO_DO_Init_s  Parameters=SampleTime,do_channel,diagnostic,safety_conf  SFunctionDeploymentMode=off  EnableBusSupport=off
  ErrorCode : Outport  VectorParamsAs1DForOutWhenUnconnected=off
  wires:
  IO_DO_Init_s/1 -> ErrorCode/1

== system IOBlock_Library_TTC580/DIO Blocks TTC580 IOlib/Set_DO_HighSide_Fullfb/IO_DO_ResetProtection ==
  Trigger : TriggerPort  VariantControl=(inherit)
  IO_DO_ResetProtection_s : S-Function  FunctionName=IO_DO_ResetProtection_s  Parameters=SampleTime,do_channel  SFunctionDeploymentMode=off  EnableBusSupport=off
  ErrorCode : Outport  VectorParamsAs1DForOutWhenUnconnected=off
  reset_cnt : Outport  Port=2  VectorParamsAs1DForOutWhenUnconnected=off
  wires:
  IO_DO_ResetProtection_s/1 -> ErrorCode/1
  IO_DO_ResetProtection_s/2 -> reset_cnt/1

== system IOBlock_Library_TTC580/DIO Blocks TTC580 IOlib/Set_DO_HighSide_Fullfb/IO_DO_Set ==
  do_value : Inport
  IO_DO_Set_s : S-Function  FunctionName=IO_DO_Set_s  Parameters=SampleTime,do_channel  SFunctionDeploymentMode=off  EnableBusSupport=off
  ErrorCode : Outport  VectorParamsAs1DForOutWhenUnconnected=off
  wires:
  do_value/1 -> IO_DO_Set_s/1
  IO_DO_Set_s/1 -> ErrorCode/1

== system IOBlock_Library_TTC580/DIO Blocks TTC580 IOlib/Set_DO_HighSide_Fullfb/compare2FET_PROT_REENABLE ==
  Errorcode : Inport  OutDataTypeStr=uint16
  compare2error_s : S-Function  FunctionName=compare2error_s  Parameters=SampleTime,define  SFunctionDeploymentMode=off  EnableBusSupport=off
  b_compare : Outport  VectorParamsAs1DForOutWhenUnconnected=off
  wires:
  Errorcode/1 -> compare2error_s/1
  compare2error_s/1 -> b_compare/1

== system IOBlock_Library_TTC580/DIO Blocks TTC580 IOlib/Set_DO_LowSide/IO_DO_Init ==
  IO_DO_Init_s : S-Function  FunctionName=IO_DO_Init_s  Parameters=SampleTime,do_channel,diagnostic,safety_conf  SFunctionDeploymentMode=off  EnableBusSupport=off
  ErrorCode : Outport  VectorParamsAs1DForOutWhenUnconnected=off
  wires:
  IO_DO_Init_s/1 -> ErrorCode/1

== system IOBlock_Library_TTC580/DIO Blocks TTC580 IOlib/Set_DO_LowSide/IO_DO_ResetProtection ==
  Trigger : TriggerPort  VariantControl=(inherit)
  IO_DO_ResetProtection_s : S-Function  FunctionName=IO_DO_ResetProtection_s  Parameters=SampleTime,do_channel  SFunctionDeploymentMode=off  EnableBusSupport=off
  ErrorCode : Outport  VectorParamsAs1DForOutWhenUnconnected=off
  reset_cnt : Outport  Port=2  VectorParamsAs1DForOutWhenUnconnected=off
  wires:
  IO_DO_ResetProtection_s/1 -> ErrorCode/1
  IO_DO_ResetProtection_s/2 -> reset_cnt/1

== system IOBlock_Library_TTC580/DIO Blocks TTC580 IOlib/Set_DO_LowSide/IO_DO_Set ==
  do_value : Inport
  IO_DO_Set_s : S-Function  FunctionName=IO_DO_Set_s  Parameters=SampleTime,do_channel  SFunctionDeploymentMode=off  EnableBusSupport=off
  ErrorCode : Outport  VectorParamsAs1DForOutWhenUnconnected=off
  wires:
  do_value/1 -> IO_DO_Set_s/1
  IO_DO_Set_s/1 -> ErrorCode/1

== system IOBlock_Library_TTC580/DIO Blocks TTC580 IOlib/Set_DO_LowSide/compare2FET_PROT_REENABLE ==
  Errorcode : Inport  OutDataTypeStr=uint16
  compare2error_s : S-Function  FunctionName=compare2error_s  Parameters=SampleTime,define  SFunctionDeploymentMode=off  EnableBusSupport=off
  b_compare : Outport  VectorParamsAs1DForOutWhenUnconnected=off
  wires:
  Errorcode/1 -> compare2error_s/1
  compare2error_s/1 -> b_compare/1

== system IOBlock_Library_TTC580/EEPROM Blocks TTC580 IOlib/CRC32_EEPROM_Read/EEPROM_Mirror ==
  EC_EEPROM_Init : Inport
  EEPROM_Mirror_s : S-Function  FunctionName=EEPROM_Mirror_s  Parameters=SampleTime,offset,length  SFunctionDeploymentMode=off  EnableBusSupport=off
  Terminator : Terminator
  wires:
  EC_EEPROM_Init/1 -> EEPROM_Mirror_s/1
  EEPROM_Mirror_s/1 -> Terminator/1

== system IOBlock_Library_TTC580/EEPROM Blocks TTC580 IOlib/CRC32_EEPROM_Read/IO_EEPROM_GetStatus ==
  IO_EEPROM_GetStatus_s : S-Function  FunctionName=IO_EEPROM_GetStatus_s  Parameters=SampleTime  SFunctionDeploymentMode=off  EnableBusSupport=off
  ErrorCode : Outport  VectorParamsAs1DForOutWhenUnconnected=off
  wires:
  IO_EEPROM_GetStatus_s/1 -> ErrorCode/1

== system IOBlock_Library_TTC580/EEPROM Blocks TTC580 IOlib/CRC32_EEPROM_Read/IO_EEPROM_Init ==
  IO_EEPROM_Init_s : S-Function  FunctionName=IO_EEPROM_Init_s  Parameters=SampleTime  SFunctionDeploymentMode=off  EnableBusSupport=off
  ErrorCode : Outport  VectorParamsAs1DForOutWhenUnconnected=off
  wires:
  IO_EEPROM_Init_s/1 -> ErrorCode/1

== system IOBlock_Library_TTC580/EEPROM Blocks TTC580 IOlib/CRC32_EEPROM_Read/Read_Mirror ==
  Read_Mirror_s : S-Function  FunctionName=Read_Mirror_s  Parameters=SampleTime,offset,length  SFunctionDeploymentMode=off  EnableBusSupport=off
  ErrorCode_EEPROM_mirror : Outport  VectorParamsAs1DForOutWhenUnconnected=off
  data : Outport  Port=2  VectorParamsAs1DForOutWhenUnconnected=off
  wires:
  Read_Mirror_s/1 -> ErrorCode_EEPROM_mirror/1
  Read_Mirror_s/2 -> data/1

== system IOBlock_Library_TTC580/EEPROM Blocks TTC580 IOlib/CRC32_EEPROM_Read/check & freeze ==
  check1 : Inport
  b_enable : Inport  Port=2
  check2 : Inport  Port=3
  Trigger : TriggerPort  VariantControl=(inherit)
  Logical Operator1 : Logic  AllPortsSameDT=off  OutDataTypeStr=boolean
  Relational Operator : RelationalOperator  Operator===  OutDataTypeStr=boolean  RndMeth=Nearest
  Out : Outport  InitialOutput=0  VectorParamsAs1DForOutWhenUnconnected=off
  wires:
  check2/1 -> Relational Operator/2
  b_enable/1 -> Logical Operator1/2
  Logical Operator1/1 -> Out/1
  check1/1 -> Relational Operator/1
  Relational Operator/1 -> Logical Operator1/1

== system IOBlock_Library_TTC580/EEPROM Blocks TTC580 IOlib/CRC32_EEPROM_Read/crc32_calc_intern ==
  Trigger : TriggerPort  VariantControl=(inherit)
  crc32_calc_intern_s : S-Function  FunctionName=crc32_calc_intern_s  Parameters=SampleTime,EEPROM_mirror,iBasicAddr_intern,iEndAddr_intern  SFunctionDeploymentMode=off  EnableBusSupport=off
  ErrorCode : Outport  VectorParamsAs1DForOutWhenUnconnected=off
  crc32 : Outport  Port=2  VectorParamsAs1DForOutWhenUnconnected=off
  wires:
  crc32_calc_intern_s/1 -> ErrorCode/1
  crc32_calc_intern_s/2 -> crc32/1

== system IOBlock_Library_TTC580/EEPROM Blocks TTC580 IOlib/CRC32_EEPROM_Read/once_true: Mirror filled ==
  S : Inport
  Logic : CombinatorialLogic  TruthTable=[0 ;1 ;0 ;0 ;1 ;1 ;0 ;0 ]
  Memory : Memory  InitialCondition=initial_condition  InheritSampleTime=on
  Mux : Mux  Inputs=3
  R : Constant  Value=0  OutDataTypeStr=boolean
  Q : Outport  InitialOutput=0  VectorParamsAs1DForOutWhenUnconnected=off
  wires:
  Memory/1 -> Mux/3
  Mux/1 -> Logic/1
  Logic/1 -> Q/1, Memory/1
  S/1 -> Mux/1
  R/1 -> Mux/2

== system IOBlock_Library_TTC580/EEPROM Blocks TTC580 IOlib/CRC32_EEPROM_Write/EEPROM_Mirror ==
  EC_EEPROM_Init : Inport
  EEPROM_Mirror_s : S-Function  FunctionName=EEPROM_Mirror_s  Parameters=SampleTime,offset,length  SFunctionDeploymentMode=off  EnableBusSupport=off
  Terminator : Terminator
  wires:
  EC_EEPROM_Init/1 -> EEPROM_Mirror_s/1
  EEPROM_Mirror_s/1 -> Terminator/1

== system IOBlock_Library_TTC580/EEPROM Blocks TTC580 IOlib/CRC32_EEPROM_Write/IO_EEPROM_GetStatus ==
  IO_EEPROM_GetStatus_s : S-Function  FunctionName=IO_EEPROM_GetStatus_s  Parameters=SampleTime  SFunctionDeploymentMode=off  EnableBusSupport=off
  ErrorCode : Outport  VectorParamsAs1DForOutWhenUnconnected=off
  wires:
  IO_EEPROM_GetStatus_s/1 -> ErrorCode/1

== system IOBlock_Library_TTC580/EEPROM Blocks TTC580 IOlib/CRC32_EEPROM_Write/IO_EEPROM_GetStatus2 ==
  IO_EEPROM_GetStatus_s : S-Function  FunctionName=IO_EEPROM_GetStatus_s  Parameters=SampleTime  SFunctionDeploymentMode=off  EnableBusSupport=off
  ErrorCode : Outport  VectorParamsAs1DForOutWhenUnconnected=off
  wires:
  IO_EEPROM_GetStatus_s/1 -> ErrorCode/1

== system IOBlock_Library_TTC580/EEPROM Blocks TTC580 IOlib/CRC32_EEPROM_Write/IO_EEPROM_Init ==
  IO_EEPROM_Init_s : S-Function  FunctionName=IO_EEPROM_Init_s  Parameters=SampleTime  SFunctionDeploymentMode=off  EnableBusSupport=off
  ErrorCode : Outport  VectorParamsAs1DForOutWhenUnconnected=off
  wires:
  IO_EEPROM_Init_s/1 -> ErrorCode/1

== system IOBlock_Library_TTC580/EEPROM Blocks TTC580 IOlib/CRC32_EEPROM_Write/IO_EEPROM_Write ==
  EC_Write_Mirror : Inport
  GetStatus : Inport  Port=2
  IO_EEPROM_Write_s : S-Function  FunctionName=IO_EEPROM_Write_s  Parameters=SampleTime,offset,length  SFunctionDeploymentMode=off  EnableBusSupport=off
  ErrorCode : Outport  VectorParamsAs1DForOutWhenUnconnected=off
  wires:
  IO_EEPROM_Write_s/1 -> ErrorCode/1
  GetStatus/1 -> IO_EEPROM_Write_s/2
  EC_Write_Mirror/1 -> IO_EEPROM_Write_s/1

== system IOBlock_Library_TTC580/EEPROM Blocks TTC580 IOlib/CRC32_EEPROM_Write/Write_Mirror ==
  b_trigger : Inport
  data : Inport  Port=2
  Write_Mirror_s : S-Function  FunctionName=Write_Mirror_s  Parameters=SampleTime,offset,length  SFunctionDeploymentMode=off  EnableBusSupport=off
  ErrorCode_EEPROM_mirror : Outport  VectorParamsAs1DForOutWhenUnconnected=off
  wires:
  Write_Mirror_s/1 -> ErrorCode_EEPROM_mirror/1
  data/1 -> Write_Mirror_s/2
  b_trigger/1 -> Write_Mirror_s/1

== system IOBlock_Library_TTC580/EEPROM Blocks TTC580 IOlib/CRC32_EEPROM_Write/crc32_calc_intern ==
  Trigger : TriggerPort  VariantControl=(inherit)
  crc32_calc_intern_s : S-Function  FunctionName=crc32_calc_intern_s  Parameters=SampleTime,EEPROM_mirror,iBasicAddr_intern,iEndAddr_intern  SFunctionDeploymentMode=off  EnableBusSupport=off
  ErrorCode : Outport  VectorParamsAs1DForOutWhenUnconnected=off
  crc32 : Outport  Port=2  VectorParamsAs1DForOutWhenUnconnected=off
  wires:
  crc32_calc_intern_s/1 -> ErrorCode/1
  crc32_calc_intern_s/2 -> crc32/1

== system IOBlock_Library_TTC580/EEPROM Blocks TTC580 IOlib/EEPROM_Read/EEPROM_Mirror ==
  EC_EEPROM_Init : Inport
  EEPROM_Mirror_s : S-Function  FunctionName=EEPROM_Mirror_s  Parameters=SampleTime,offset,length  SFunctionDeploymentMode=off  EnableBusSupport=off
  Terminator : Terminator
  wires:
  EEPROM_Mirror_s/1 -> Terminator/1
  EC_EEPROM_Init/1 -> EEPROM_Mirror_s/1

== system IOBlock_Library_TTC580/EEPROM Blocks TTC580 IOlib/EEPROM_Read/IO_EEPROM_GetStatus ==
  IO_EEPROM_GetStatus_s : S-Function  FunctionName=IO_EEPROM_GetStatus_s  Parameters=SampleTime  SFunctionDeploymentMode=off  EnableBusSupport=off
  ErrorCode : Outport  VectorParamsAs1DForOutWhenUnconnected=off
  wires:
  IO_EEPROM_GetStatus_s/1 -> ErrorCode/1

== system IOBlock_Library_TTC580/EEPROM Blocks TTC580 IOlib/EEPROM_Read/IO_EEPROM_Init ==
  IO_EEPROM_Init_s : S-Function  FunctionName=IO_EEPROM_Init_s  Parameters=SampleTime  SFunctionDeploymentMode=off  EnableBusSupport=off
  ErrorCode : Outport  VectorParamsAs1DForOutWhenUnconnected=off
  wires:
  IO_EEPROM_Init_s/1 -> ErrorCode/1

== system IOBlock_Library_TTC580/EEPROM Blocks TTC580 IOlib/EEPROM_Read/Read_Mirror ==
  Read_Mirror_s : S-Function  FunctionName=Read_Mirror_s  Parameters=SampleTime,offset,length  SFunctionDeploymentMode=off  EnableBusSupport=off
  ErrorCode_EEPROM_mirror : Outport  VectorParamsAs1DForOutWhenUnconnected=off
  data : Outport  Port=2  VectorParamsAs1DForOutWhenUnconnected=off
  wires:
  Read_Mirror_s/1 -> ErrorCode_EEPROM_mirror/1
  Read_Mirror_s/2 -> data/1

== system IOBlock_Library_TTC580/EEPROM Blocks TTC580 IOlib/EEPROM_Read/once_true: Mirror filled ==
  S : Inport
  Logic : CombinatorialLogic  TruthTable=[0 ;1 ;0 ;0 ;1 ;1 ;0 ;0 ]
  Memory : Memory  InitialCondition=initial_condition  InheritSampleTime=on
  Mux : Mux  Inputs=3
  R : Constant  Value=0  OutDataTypeStr=boolean
  Q : Outport  InitialOutput=0  VectorParamsAs1DForOutWhenUnconnected=off
  wires:
  Memory/1 -> Mux/3
  Mux/1 -> Logic/1
  Logic/1 -> Q/1, Memory/1
  S/1 -> Mux/1
  R/1 -> Mux/2

== system IOBlock_Library_TTC580/EEPROM Blocks TTC580 IOlib/EEPROM_Read_OffsetIn/EEPROM_Mirror ==
  EC_EEPROM_Init : Inport
  EEPROM_Mirror_s : S-Function  FunctionName=EEPROM_Mirror_s  Parameters=SampleTime,offset,length  SFunctionDeploymentMode=off  EnableBusSupport=off
  Terminator : Terminator
  wires:
  EEPROM_Mirror_s/1 -> Terminator/1
  EC_EEPROM_Init/1 -> EEPROM_Mirror_s/1

== system IOBlock_Library_TTC580/EEPROM Blocks TTC580 IOlib/EEPROM_Read_OffsetIn/IO_EEPROM_GetStatus ==
  IO_EEPROM_GetStatus_s : S-Function  FunctionName=IO_EEPROM_GetStatus_s  Parameters=SampleTime  SFunctionDeploymentMode=off  EnableBusSupport=off
  ErrorCode : Outport  VectorParamsAs1DForOutWhenUnconnected=off
  wires:
  IO_EEPROM_GetStatus_s/1 -> ErrorCode/1

== system IOBlock_Library_TTC580/EEPROM Blocks TTC580 IOlib/EEPROM_Read_OffsetIn/IO_EEPROM_Init ==
  IO_EEPROM_Init_s : S-Function  FunctionName=IO_EEPROM_Init_s  Parameters=SampleTime  SFunctionDeploymentMode=off  EnableBusSupport=off
  ErrorCode : Outport  VectorParamsAs1DForOutWhenUnconnected=off
  wires:
  IO_EEPROM_Init_s/1 -> ErrorCode/1

== system IOBlock_Library_TTC580/EEPROM Blocks TTC580 IOlib/EEPROM_Read_OffsetIn/Read_Mirror_OffsetIn ==
  offset : Inport
  Read_Mirror_OffsetIn_s : S-Function  FunctionName=Read_Mirror_OffsetIn_s  Parameters=SampleTime,length  SFunctionDeploymentMode=off  EnableBusSupport=off
  ErrorCode_EEPROM_mirror : Outport  VectorParamsAs1DForOutWhenUnconnected=off
  data : Outport  Port=2  VectorParamsAs1DForOutWhenUnconnected=off
  wires:
  Read_Mirror_OffsetIn_s/2 -> data/1
  Read_Mirror_OffsetIn_s/1 -> ErrorCode_EEPROM_mirror/1
  offset/1 -> Read_Mirror_OffsetIn_s/1

== system IOBlock_Library_TTC580/EEPROM Blocks TTC580 IOlib/EEPROM_Read_OffsetIn/once_true: Mirror filled ==
  S : Inport
  Logic : CombinatorialLogic  TruthTable=[0 ;1 ;0 ;0 ;1 ;1 ;0 ;0 ]
  Memory : Memory  InitialCondition=initial_condition  InheritSampleTime=on
  Mux : Mux  Inputs=3
  R : Constant  Value=0  OutDataTypeStr=boolean
  Q : Outport  InitialOutput=0  VectorParamsAs1DForOutWhenUnconnected=off
  wires:
  Memory/1 -> Mux/3
  Mux/1 -> Logic/1
  Logic/1 -> Q/1, Memory/1
  S/1 -> Mux/1
  R/1 -> Mux/2

== system IOBlock_Library_TTC580/EEPROM Blocks TTC580 IOlib/EEPROM_Read_Raw/IO_EEPROM_Init ==
  IO_EEPROM_Init_s : S-Function  FunctionName=IO_EEPROM_Init_s  Parameters=SampleTime  SFunctionDeploymentMode=off  EnableBusSupport=off
  ErrorCode : Outport  VectorParamsAs1DForOutWhenUnconnected=off
  wires:
  IO_EEPROM_Init_s/1 -> ErrorCode/1

== system IOBlock_Library_TTC580/EEPROM Blocks TTC580 IOlib/EEPROM_Read_Raw/IO_EEPROM_Read_raw ==
  IO_EEPROM_Read_raw_s : S-Function  FunctionName=IO_EEPROM_Read_raw_s  Parameters=SampleTime,offset,length  SFunctionDeploymentMode=off  EnableBusSupport=off
  ErrorCode : Outport  VectorParamsAs1DForOutWhenUnconnected=off
  data : Outport  Port=2  VectorParamsAs1DForOutWhenUnconnected=off
  wires:
  IO_EEPROM_Read_raw_s/2 -> data/1
  IO_EEPROM_Read_raw_s/1 -> ErrorCode/1

== system IOBlock_Library_TTC580/EEPROM Blocks TTC580 IOlib/EEPROM_Write/EEPROM_Mirror ==
  EC_EEPROM_Init : Inport
  EEPROM_Mirror_s : S-Function  FunctionName=EEPROM_Mirror_s  Parameters=SampleTime,offset,length  SFunctionDeploymentMode=off  EnableBusSupport=off
  Terminator : Terminator
  wires:
  EEPROM_Mirror_s/1 -> Terminator/1
  EC_EEPROM_Init/1 -> EEPROM_Mirror_s/1

== system IOBlock_Library_TTC580/EEPROM Blocks TTC580 IOlib/EEPROM_Write/IO_EEPROM_GetStatus ==
  IO_EEPROM_GetStatus_s : S-Function  FunctionName=IO_EEPROM_GetStatus_s  Parameters=SampleTime  SFunctionDeploymentMode=off  EnableBusSupport=off
  ErrorCode : Outport  VectorParamsAs1DForOutWhenUnconnected=off
  wires:
  IO_EEPROM_GetStatus_s/1 -> ErrorCode/1

== system IOBlock_Library_TTC580/EEPROM Blocks TTC580 IOlib/EEPROM_Write/IO_EEPROM_GetStatus1 ==
  IO_EEPROM_GetStatus_s : S-Function  FunctionName=IO_EEPROM_GetStatus_s  Parameters=SampleTime  SFunctionDeploymentMode=off  EnableBusSupport=off
  ErrorCode : Outport  VectorParamsAs1DForOutWhenUnconnected=off
  wires:
  IO_EEPROM_GetStatus_s/1 -> ErrorCode/1

== system IOBlock_Library_TTC580/EEPROM Blocks TTC580 IOlib/EEPROM_Write/IO_EEPROM_Init ==
  IO_EEPROM_Init_s : S-Function  FunctionName=IO_EEPROM_Init_s  Parameters=SampleTime  SFunctionDeploymentMode=off  EnableBusSupport=off
  ErrorCode : Outport  VectorParamsAs1DForOutWhenUnconnected=off
  wires:
  IO_EEPROM_Init_s/1 -> ErrorCode/1
